simulink library "roller485lib"  (R2023a)
settings: Solver=VariableStepAuto  StartTime=0.0  StopTime=10.0  RelTol=1e-3
libraries: arduinolib x172, simulink x66, $bdroot x1
(part 3 of 5)

== system roller485lib/I2C Write/current command [A] ==
  command [A] : Inport
  A to mA : Gain  Gain=1000
  "Clock " : Clock
  Compare To Constant : simulink/Logic and Bit Operations/Compare To Constant  relop=<=  const=set_time  OutDataTypeStr=boolean
  Data Type Conversion : DataTypeConversion  OutDataTypeStr=uint32  SaturateOnIntegerOverflow=off  RndMeth=Floor
  Enabled Subsystem (mode setting) : $bdroot/I2C Write/current command [mA]/Enabled Subsystem (mode setting)  SystemSampleTime=-1  VariantActivationTime=update diagram  Latency=0  AutoFrameSizeCalculation=off
  I2C Write (0xB0) : arduinolib/I2C Write  I2CModule=0  Mode=Master  SlaveAddress=I2CAddress  SlaveByteOrder=LittleEndian  Direction=Transmitter  RegisterAddressMode=on  RegisterAddress=0xB0  SlaveDataType=uint8  DataLength=1  NoAck=off  RepeatedStart=off  OutputStatus=off  blockPlatform=ARDUINO
  current mode : Constant  Value=3
  x 100 : Gain  Gain=100
  wires:
  x 100/1 -> Data Type Conversion/1
  command [A]/1 -> A to mA/1
  A to mA/1 -> x 100/1
  Data Type Conversion/1 -> I2C Write (0xB0)/1
  Compare To Constant/1 -> Enabled Subsystem (mode setting)/Enable
  current mode/1 -> Enabled Subsystem (mode setting)/1
  "Clock "/1 -> Compare To Constant/1

== system roller485lib/I2C Write/current command [mA] ==
  command [mA] : Inport
  "Clock " : Clock
  Compare To Constant : simulink/Logic and Bit Operations/Compare To Constant  relop=<=  const=set_time  OutDataTypeStr=boolean
  Data Type Conversion : DataTypeConversion  OutDataTypeStr=uint32  SaturateOnIntegerOverflow=off  RndMeth=Floor
  Enabled Subsystem (mode setting) : Subsystem  TreatAsAtomicUnit=on
  I2C Write (0xB0) : arduinolib/I2C Write  I2CModule=0  Mode=Master  SlaveAddress=I2CAddress  SlaveByteOrder=LittleEndian  Direction=Transmitter  RegisterAddressMode=on  RegisterAddress=0xB0  SlaveDataType=uint8  DataLength=1  NoAck=off  RepeatedStart=off  OutputStatus=off  blockPlatform=ARDUINO
  current mode : Constant  Value=3
  x 100 : Gain  Gain=100
  wires:
  current mode/1 -> Enabled Subsystem (mode setting)/1(mode)
  Compare To Constant/1 -> Enabled Subsystem (mode setting)/Enable
  "Clock "/1 -> Compare To Constant/1
  Data Type Conversion/1 -> I2C Write (0xB0)/1
  command [mA]/1 -> x 100/1
  x 100/1 -> Data Type Conversion/1

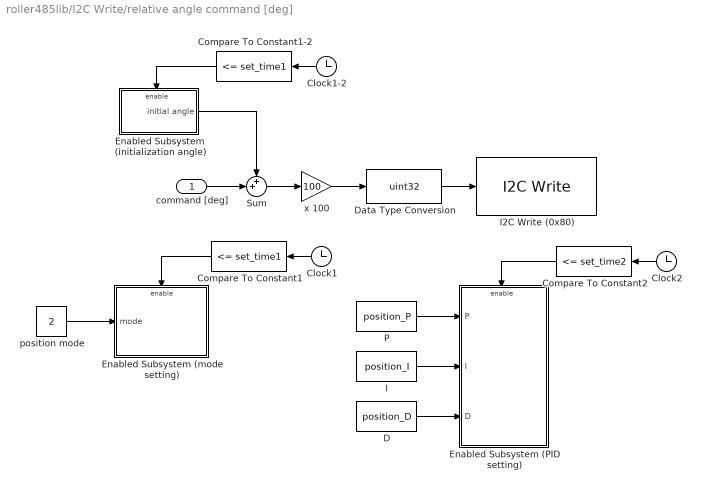
== system roller485lib/I2C Write/relative angle command [deg] ==
  command [deg] : Inport
  Clock1 : Clock
  Clock1-2 : Clock
  Clock2 : Clock
  Compare To Constant1 : simulink/Logic and Bit Operations/Compare To Constant  relop=<=  const=set_time1  OutDataTypeStr=boolean
  Compare To Constant1-2 : simulink/Logic and Bit Operations/Compare To Constant  relop=<=  const=set_time1  OutDataTypeStr=boolean
  Compare To Constant2 : simulink/Logic and Bit Operations/Compare To Constant  relop=<=  const=set_time2  OutDataTypeStr=boolean
  D : Constant  Value=position_D
  Data Type Conversion : DataTypeConversion  OutDataTypeStr=uint32  SaturateOnIntegerOverflow=off  RndMeth=Floor
  Enabled Subsystem (PID setting) : Subsystem  TreatAsAtomicUnit=on
  Enabled Subsystem (initialization angle) : Subsystem  TreatAsAtomicUnit=on
  Enabled Subsystem (mode setting) : Subsystem  TreatAsAtomicUnit=on
  I : Constant  Value=position_I
  I2C Write (0x80) : arduinolib/I2C Write  I2CModule=0  Mode=Master  SlaveAddress=I2CAddress  SlaveByteOrder=LittleEndian  Direction=Transmitter  RegisterAddressMode=on  RegisterAddress=0x80  SlaveDataType=uint8  DataLength=1  NoAck=off  RepeatedStart=off  OutputStatus=off  blockPlatform=ARDUINO
  P : Constant  Value=position_P
  Sum : Sum  Inputs=++|
  position mode : Constant  Value=2
  x 100 : Gain  Gain=100
  wires:
  Compare To Constant1-2/1 -> Enabled Subsystem (initialization angle)/Enable
  command [deg]/1 -> Sum/2
  Enabled Subsystem (initialization angle)/1(initial angle) -> Sum/1
  x 100/1 -> Data Type Conversion/1
  Sum/1 -> x 100/1
  Compare To Constant2/1 -> Enabled Subsystem (PID setting)/Enable
  position mode/1 -> Enabled Subsystem (mode setting)/1(mode)
  P/1 -> Enabled Subsystem (PID setting)/1(P)
  Clock1/1 -> Compare To Constant1/1
  Compare To Constant1/1 -> Enabled Subsystem (mode setting)/Enable
  Data Type Conversion/1 -> I2C Write (0x80)/1
  D/1 -> Enabled Subsystem (PID setting)/3(D)
  I/1 -> Enabled Subsystem (PID setting)/2(I)
  Clock2/1 -> Compare To Constant2/1
  Clock1-2/1 -> Compare To Constant1-2/1

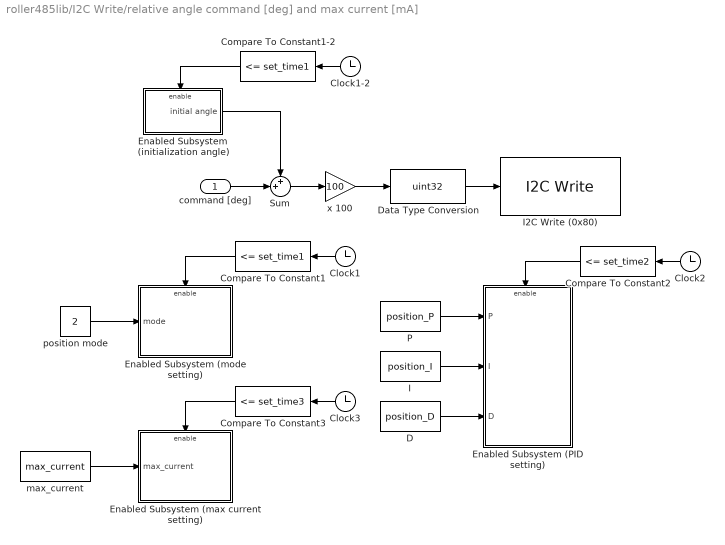
== system roller485lib/I2C Write/relative angle command [deg] and max current [mA] ==
  command [deg] : Inport
  Clock1 : Clock
  Clock1-2 : Clock
  Clock2 : Clock
  Clock3 : Clock
  Compare To Constant1 : simulink/Logic and Bit Operations/Compare To Constant  relop=<=  const=set_time1  OutDataTypeStr=boolean
  Compare To Constant1-2 : simulink/Logic and Bit Operations/Compare To Constant  relop=<=  const=set_time1  OutDataTypeStr=boolean
  Compare To Constant2 : simulink/Logic and Bit Operations/Compare To Constant  relop=<=  const=set_time2  OutDataTypeStr=boolean
  Compare To Constant3 : simulink/Logic and Bit Operations/Compare To Constant  relop=<=  const=set_time3  OutDataTypeStr=boolean
  D : Constant  Value=position_D
  Data Type Conversion : DataTypeConversion  OutDataTypeStr=uint32  SaturateOnIntegerOverflow=off  RndMeth=Floor
  Enabled Subsystem (PID setting) : Subsystem  TreatAsAtomicUnit=on
  Enabled Subsystem (initialization angle) : Subsystem  TreatAsAtomicUnit=on
  Enabled Subsystem (max current setting) : Subsystem  TreatAsAtomicUnit=on
  Enabled Subsystem (mode setting) : Subsystem  TreatAsAtomicUnit=on
  I : Constant  Value=position_I
  I2C Write (0x80) : arduinolib/I2C Write  I2CModule=0  Mode=Master  SlaveAddress=I2CAddress  SlaveByteOrder=LittleEndian  Direction=Transmitter  RegisterAddressMode=on  RegisterAddress=0x80  SlaveDataType=uint8  DataLength=1  NoAck=off  RepeatedStart=off  OutputStatus=off  blockPlatform=ARDUINO
  P : Constant  Value=position_P
  Sum : Sum  Inputs=++|
  max_current : Constant  Value=max_current
  position mode : Constant  Value=2
  x 100 : Gain  Gain=100
  wires:
  Compare To Constant1-2/1 -> Enabled Subsystem (initialization angle)/Enable
  command [deg]/1 -> Sum/2
  Enabled Subsystem (initialization angle)/1(initial angle) -> Sum/1
  x 100/1 -> Data Type Conversion/1
  Sum/1 -> x 100/1
  max_current/1 -> Enabled Subsystem (max current setting)/1(max_current)
  Compare To Constant2/1 -> Enabled Subsystem (PID setting)/Enable
  Compare To Constant3/1 -> Enabled Subsystem (max current setting)/Enable
  position mode/1 -> Enabled Subsystem (mode setting)/1(mode)
  P/1 -> Enabled Subsystem (PID setting)/1(P)
  Clock1/1 -> Compare To Constant1/1
  Compare To Constant1/1 -> Enabled Subsystem (mode setting)/Enable
  Data Type Conversion/1 -> I2C Write (0x80)/1
  D/1 -> Enabled Subsystem (PID setting)/3(D)
  I/1 -> Enabled Subsystem (PID setting)/2(I)
  Clock3/1 -> Compare To Constant3/1
  Clock2/1 -> Compare To Constant2/1
  Clock1-2/1 -> Compare To Constant1-2/1

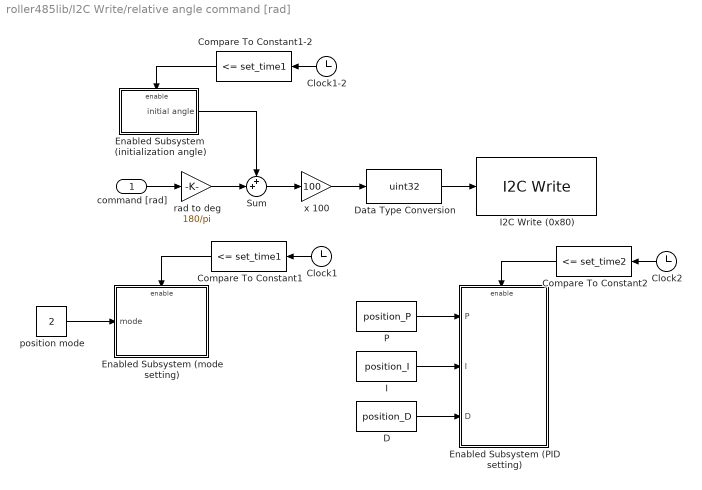
== system roller485lib/I2C Write/relative angle command [rad] ==
  command [rad] : Inport
  Clock1 : Clock
  Clock1-2 : Clock
  Clock2 : Clock
  Compare To Constant1 : simulink/Logic and Bit Operations/Compare To Constant  relop=<=  const=set_time1  OutDataTypeStr=boolean
  Compare To Constant1-2 : simulink/Logic and Bit Operations/Compare To Constant  relop=<=  const=set_time1  OutDataTypeStr=boolean
  Compare To Constant2 : simulink/Logic and Bit Operations/Compare To Constant  relop=<=  const=set_time2  OutDataTypeStr=boolean
  D : Constant  Value=position_D
  Data Type Conversion : DataTypeConversion  OutDataTypeStr=uint32  SaturateOnIntegerOverflow=off  RndMeth=Floor
  Enabled Subsystem (PID setting) : Subsystem  TreatAsAtomicUnit=on
  Enabled Subsystem (initialization angle) : Subsystem  TreatAsAtomicUnit=on
  Enabled Subsystem (mode setting) : Subsystem  TreatAsAtomicUnit=on
  I : Constant  Value=position_I
  I2C Write (0x80) : arduinolib/I2C Write  I2CModule=0  Mode=Master  SlaveAddress=I2CAddress  SlaveByteOrder=LittleEndian  Direction=Transmitter  RegisterAddressMode=on  RegisterAddress=0x80  SlaveDataType=uint8  DataLength=1  NoAck=off  RepeatedStart=off  OutputStatus=off  blockPlatform=ARDUINO
  P : Constant  Value=position_P
  Sum : Sum  Inputs=++|
  position mode : Constant  Value=2
  rad to deg : Gain  Gain=180/pi
  x 100 : Gain  Gain=100
  wires:
  Compare To Constant1-2/1 -> Enabled Subsystem (initialization angle)/Enable
  command [rad]/1 -> rad to deg/1
  rad to deg/1 -> Sum/2
  Enabled Subsystem (initialization angle)/1(initial angle) -> Sum/1
  x 100/1 -> Data Type Conversion/1
  Sum/1 -> x 100/1
  Compare To Constant2/1 -> Enabled Subsystem (PID setting)/Enable
  position mode/1 -> Enabled Subsystem (mode setting)/1(mode)
  P/1 -> Enabled Subsystem (PID setting)/1(P)
  Clock1/1 -> Compare To Constant1/1
  Compare To Constant1/1 -> Enabled Subsystem (mode setting)/Enable
  Data Type Conversion/1 -> I2C Write (0x80)/1
  D/1 -> Enabled Subsystem (PID setting)/3(D)
  I/1 -> Enabled Subsystem (PID setting)/2(I)
  Clock2/1 -> Compare To Constant2/1
  Clock1-2/1 -> Compare To Constant1-2/1

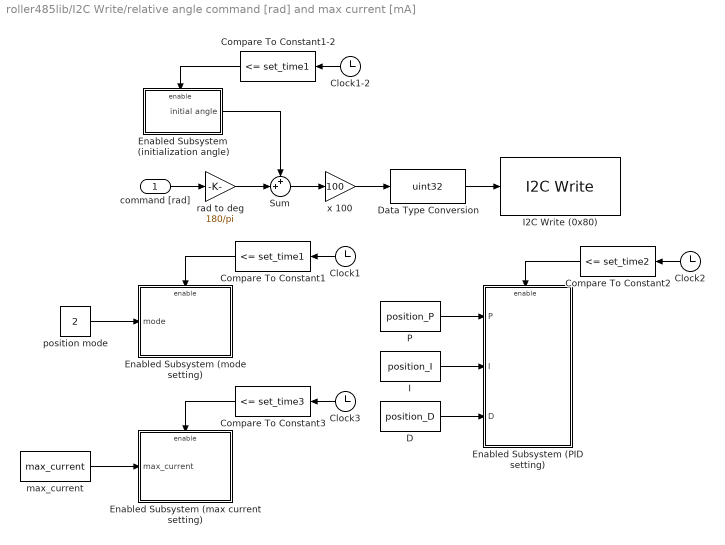
== system roller485lib/I2C Write/relative angle command [rad] and max current [mA] ==
  command [rad] : Inport
  Clock1 : Clock
  Clock1-2 : Clock
  Clock2 : Clock
  Clock3 : Clock
  Compare To Constant1 : simulink/Logic and Bit Operations/Compare To Constant  relop=<=  const=set_time1  OutDataTypeStr=boolean
  Compare To Constant1-2 : simulink/Logic and Bit Operations/Compare To Constant  relop=<=  const=set_time1  OutDataTypeStr=boolean
  Compare To Constant2 : simulink/Logic and Bit Operations/Compare To Constant  relop=<=  const=set_time2  OutDataTypeStr=boolean
  Compare To Constant3 : simulink/Logic and Bit Operations/Compare To Constant  relop=<=  const=set_time3  OutDataTypeStr=boolean
  D : Constant  Value=position_D
  Data Type Conversion : DataTypeConversion  OutDataTypeStr=uint32  SaturateOnIntegerOverflow=off  RndMeth=Floor
  Enabled Subsystem (PID setting) : Subsystem  TreatAsAtomicUnit=on
  Enabled Subsystem (initialization angle) : Subsystem  TreatAsAtomicUnit=on
  Enabled Subsystem (max current setting) : Subsystem  TreatAsAtomicUnit=on
  Enabled Subsystem (mode setting) : Subsystem  TreatAsAtomicUnit=on
  I : Constant  Value=position_I
  I2C Write (0x80) : arduinolib/I2C Write  I2CModule=0  Mode=Master  SlaveAddress=I2CAddress  SlaveByteOrder=LittleEndian  Direction=Transmitter  RegisterAddressMode=on  RegisterAddress=0x80  SlaveDataType=uint8  DataLength=1  NoAck=off  RepeatedStart=off  OutputStatus=off  blockPlatform=ARDUINO
  P : Constant  Value=position_P
  Sum : Sum  Inputs=++|
  max_current : Constant  Value=max_current
  position mode : Constant  Value=2
  rad to deg : Gain  Gain=180/pi
  x 100 : Gain  Gain=100
  wires:
  Enabled Subsystem (initialization angle)/1(initial angle) -> Sum/1
  command [rad]/1 -> rad to deg/1
  x 100/1 -> Data Type Conversion/1
  Sum/1 -> x 100/1
  Data Type Conversion/1 -> I2C Write (0x80)/1
  rad to deg/1 -> Sum/2
  Clock2/1 -> Compare To Constant2/1
  D/1 -> Enabled Subsystem (PID setting)/3(D)
  Compare To Constant1/1 -> Enabled Subsystem (mode setting)/Enable
  I/1 -> Enabled Subsystem (PID setting)/2(I)
  Clock1/1 -> Compare To Constant1/1
  position mode/1 -> Enabled Subsystem (mode setting)/1(mode)
  Compare To Constant3/1 -> Enabled Subsystem (max current setting)/Enable
  Clock3/1 -> Compare To Constant3/1
  P/1 -> Enabled Subsystem (PID setting)/1(P)
  max_current/1 -> Enabled Subsystem (max current setting)/1(max_current)
  Compare To Constant2/1 -> Enabled Subsystem (PID setting)/Enable
  Compare To Constant1-2/1 -> Enabled Subsystem (initialization angle)/Enable
  Clock1-2/1 -> Compare To Constant1-2/1

== system roller485lib/I2C Write (using MATLAB Function)/absolute angle command [deg] (using MATLAB Function) ==
  command [deg] : Inport
  Clock1 : Clock
  Clock2 : Clock
  Compare To Constant1 : simulink/Logic and Bit Operations/Compare To Constant  relop=<=  const=set_time1  OutDataTypeStr=boolean
  Compare To Constant2 : simulink/Logic and Bit Operations/Compare To Constant  relop=<=  const=set_time2  OutDataTypeStr=boolean
  D : Constant  Value=position_D
  Enabled Subsystem (PID setting) : Subsystem  TreatAsAtomicUnit=on
  Enabled Subsystem (mode setting) : Subsystem  TreatAsAtomicUnit=on
  I : Constant  Value=position_I
  I2C Write (0x80) : arduinolib/I2C Write  I2CModule=0  Mode=Master  SlaveAddress=I2CAddress  SlaveByteOrder=BigEndian  Direction=Transmitter  RegisterAddressMode=on  RegisterAddress=0x80  SlaveDataType=uint8  DataLength=1  NoAck=off  RepeatedStart=off  OutputStatus=off  blockPlatform=ARDUINO
  MATLAB Function : MATLAB Function  TreatAsAtomicUnit=on
  P : Constant  Value=position_P
  position mode : Constant  Value=2
  x 100 : Gain  Gain=100
  wires:
  command [deg]/1 -> x 100/1
  x 100/1 -> MATLAB Function/1(double_data)
  D/1 -> Enabled Subsystem (PID setting)/3(D)
  I/1 -> Enabled Subsystem (PID setting)/2(I)
  P/1 -> Enabled Subsystem (PID setting)/1(P)
  position mode/1 -> Enabled Subsystem (mode setting)/1(mode)
  MATLAB Function/1(bytes) -> I2C Write (0x80)/1
  Compare To Constant2/1 -> Enabled Subsystem (PID setting)/Enable
  Clock1/1 -> Compare To Constant1/1
  Clock2/1 -> Compare To Constant2/1
  Compare To Constant1/1 -> Enabled Subsystem (mode setting)/Enable

== system roller485lib/I2C Write (using MATLAB Function)/absolute angle command [rad] (using MATLAB Function) ==
  command [rad] : Inport
  Clock1 : Clock
  Clock2 : Clock
  Compare To Constant1 : simulink/Logic and Bit Operations/Compare To Constant  relop=<=  const=set_time1  OutDataTypeStr=boolean
  Compare To Constant2 : simulink/Logic and Bit Operations/Compare To Constant  relop=<=  const=set_time2  OutDataTypeStr=boolean
  D : Constant  Value=position_D
  Enabled Subsystem (PID setting) : Subsystem  TreatAsAtomicUnit=on
  Enabled Subsystem (mode setting) : Subsystem  TreatAsAtomicUnit=on
  I : Constant  Value=position_I
  I2C Write (0x80) : arduinolib/I2C Write  I2CModule=0  Mode=Master  SlaveAddress=I2CAddress  SlaveByteOrder=BigEndian  Direction=Transmitter  RegisterAddressMode=on  RegisterAddress=0x80  SlaveDataType=uint8  DataLength=1  NoAck=off  RepeatedStart=off  OutputStatus=off  blockPlatform=ARDUINO
  MATLAB Function : MATLAB Function  TreatAsAtomicUnit=on
  P : Constant  Value=position_P
  position mode : Constant  Value=2
  rad to deg : Gain  Gain=180/pi
  x 100 : Gain  Gain=100
  wires:
  position mode/1 -> Enabled Subsystem (mode setting)/1(mode)
  P/1 -> Enabled Subsystem (PID setting)/1(P)
  I/1 -> Enabled Subsystem (PID setting)/2(I)
  D/1 -> Enabled Subsystem (PID setting)/3(D)
  x 100/1 -> MATLAB Function/1(double_data)
  rad to deg/1 -> x 100/1
  command [rad]/1 -> rad to deg/1
  MATLAB Function/1(bytes) -> I2C Write (0x80)/1
  Compare To Constant2/1 -> Enabled Subsystem (PID setting)/Enable
  Clock1/1 -> Compare To Constant1/1
  Clock2/1 -> Compare To Constant2/1
  Compare To Constant1/1 -> Enabled Subsystem (mode setting)/Enable

== system roller485lib/I2C Write (using MATLAB Function)/angular velocity command [rad//s] (using MATLAB Function) ==
  command [rad/s] : Inport
  Clock1 : Clock
  Clock2 : Clock
  Compare To Constant1 : simulink/Logic and Bit Operations/Compare To Constant  relop=<=  const=set_time1  OutDataTypeStr=boolean
  Compare To Constant2 : simulink/Logic and Bit Operations/Compare To Constant  relop=<=  const=set_time2  OutDataTypeStr=boolean
  D : Constant  Value=speed_D
  Enabled Subsystem (PID setting) : Subsystem  TreatAsAtomicUnit=on
  Enabled Subsystem (mode setting) : Subsystem  TreatAsAtomicUnit=on
  I : Constant  Value=speed_I
  I2C Write (0x40) : arduinolib/I2C Write  I2CModule=0  Mode=Master  SlaveAddress=I2CAddress  SlaveByteOrder=BigEndian  Direction=Transmitter  RegisterAddressMode=on  RegisterAddress=0x40  SlaveDataType=uint8  DataLength=1  NoAck=off  RepeatedStart=off  OutputStatus=off  blockPlatform=ARDUINO
  MATLAB Function : MATLAB Function  TreatAsAtomicUnit=on
  P : Constant  Value=speed_P
  rad/s to rpm : Gain  Gain=60/(2*pi)
  speed mode : Constant
  x 100 : Gain  Gain=100
  wires:
  D/1 -> Enabled Subsystem (PID setting)/3(D)
  speed mode/1 -> Enabled Subsystem (mode setting)/1(mode)
  P/1 -> Enabled Subsystem (PID setting)/1(P)
  I/1 -> Enabled Subsystem (PID setting)/2(I)
  x 100/1 -> MATLAB Function/1(double_data)
  rad/s to rpm/1 -> x 100/1
  command [rad/s]/1 -> rad/s to rpm/1
  MATLAB Function/1(bytes) -> I2C Write (0x40)/1
  Compare To Constant2/1 -> Enabled Subsystem (PID setting)/Enable
  Clock1/1 -> Compare To Constant1/1
  Clock2/1 -> Compare To Constant2/1
  Compare To Constant1/1 -> Enabled Subsystem (mode setting)/Enable

== system roller485lib/I2C Write (using MATLAB Function)/angular velocity command [rpm] (using MATLAB Function) ==
  command [rpm] : Inport
  Clock1 : Clock
  Clock2 : Clock
  Compare To Constant1 : simulink/Logic and Bit Operations/Compare To Constant  relop=<=  const=set_time1  OutDataTypeStr=boolean
  Compare To Constant2 : simulink/Logic and Bit Operations/Compare To Constant  relop=<=  const=set_time2  OutDataTypeStr=boolean
  D : Constant  Value=speed_D
  Enabled Subsystem (PID setting) : Subsystem  TreatAsAtomicUnit=on
  Enabled Subsystem (mode setting) : Subsystem  TreatAsAtomicUnit=on
  I : Constant  Value=speed_I
  I2C Write (0x40) : arduinolib/I2C Write  I2CModule=0  Mode=Master  SlaveAddress=I2CAddress  SlaveByteOrder=BigEndian  Direction=Transmitter  RegisterAddressMode=on  RegisterAddress=0x40  SlaveDataType=uint8  DataLength=1  NoAck=off  RepeatedStart=off  OutputStatus=off  blockPlatform=ARDUINO
  MATLAB Function : MATLAB Function  TreatAsAtomicUnit=on
  P : Constant  Value=speed_P
  speed mode : Constant
  x 100 : Gain  Gain=100
  wires:
  command [rpm]/1 -> x 100/1
  x 100/1 -> MATLAB Function/1(double_data)
  I/1 -> Enabled Subsystem (PID setting)/2(I)
  P/1 -> Enabled Subsystem (PID setting)/1(P)
  speed mode/1 -> Enabled Subsystem (mode setting)/1(mode)
  D/1 -> Enabled Subsystem (PID setting)/3(D)
  MATLAB Function/1(bytes) -> I2C Write (0x40)/1
  Compare To Constant2/1 -> Enabled Subsystem (PID setting)/Enable
  Clock1/1 -> Compare To Constant1/1
  Clock2/1 -> Compare To Constant2/1
  Compare To Constant1/1 -> Enabled Subsystem (mode setting)/Enable

== system roller485lib/I2C Write (using MATLAB Function)/current command [A] (using MATLAB Function) ==
  command [A] : Inport
  A to mA : Gain  Gain=1000
  "Clock " : Clock
  Compare To Constant : simulink/Logic and Bit Operations/Compare To Constant  relop=<=  const=set_time  OutDataTypeStr=boolean
  Enabled Subsystem (mode setting) : Subsystem  TreatAsAtomicUnit=on
  I2C Write (0xB0) : arduinolib/I2C Write  I2CModule=0  Mode=Master  SlaveAddress=I2CAddress  SlaveByteOrder=BigEndian  Direction=Transmitter  RegisterAddressMode=on  RegisterAddress=0xB0  SlaveDataType=uint8  DataLength=1  NoAck=off  RepeatedStart=off  OutputStatus=off  blockPlatform=ARDUINO
  MATLAB Function : MATLAB Function  TreatAsAtomicUnit=on
  current mode : Constant  Value=3
  x 100 : Gain  Gain=100
  wires:
  current mode/1 -> Enabled Subsystem (mode setting)/1(mode)
  A to mA/1 -> x 100/1
  command [A]/1 -> A to mA/1
  x 100/1 -> MATLAB Function/1(double_data)
  MATLAB Function/1(bytes) -> I2C Write (0xB0)/1
  Compare To Constant/1 -> Enabled Subsystem (mode setting)/Enable
  "Clock "/1 -> Compare To Constant/1

== system roller485lib/I2C Write (using MATLAB Function)/current command [mA] (using MATLAB Function) ==
  command [mA] : Inport
  "Clock " : Clock
  Compare To Constant : simulink/Logic and Bit Operations/Compare To Constant  relop=<=  const=set_time  OutDataTypeStr=boolean
  Enabled Subsystem (mode setting) : Subsystem  TreatAsAtomicUnit=on
  I2C Write (0xB0) : arduinolib/I2C Write  I2CModule=0  Mode=Master  SlaveAddress=I2CAddress  SlaveByteOrder=BigEndian  Direction=Transmitter  RegisterAddressMode=on  RegisterAddress=0xB0  SlaveDataType=uint8  DataLength=1  NoAck=off  RepeatedStart=off  OutputStatus=off  blockPlatform=ARDUINO
  MATLAB Function : MATLAB Function  TreatAsAtomicUnit=on
  current mode : Constant  Value=3
  x 100 : Gain  Gain=100
  wires:
  x 100/1 -> MATLAB Function/1(double_data)
  command [mA]/1 -> x 100/1
  current mode/1 -> Enabled Subsystem (mode setting)/1(mode)
  MATLAB Function/1(bytes) -> I2C Write (0xB0)/1
  Compare To Constant/1 -> Enabled Subsystem (mode setting)/Enable
  "Clock "/1 -> Compare To Constant/1

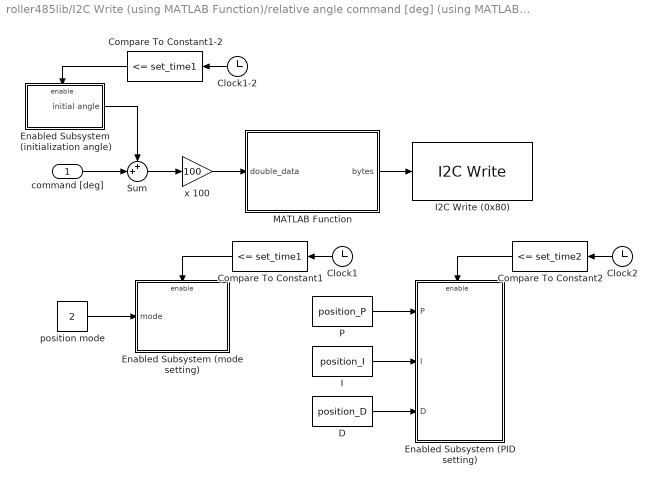
== system roller485lib/I2C Write (using MATLAB Function)/relative angle command [deg] (using MATLAB Function) ==
  command [deg] : Inport
  Clock1 : Clock
  Clock1-2 : Clock
  Clock2 : Clock
  Compare To Constant1 : simulink/Logic and Bit Operations/Compare To Constant  relop=<=  const=set_time1  OutDataTypeStr=boolean
  Compare To Constant1-2 : simulink/Logic and Bit Operations/Compare To Constant  relop=<=  const=set_time1  OutDataTypeStr=boolean
  Compare To Constant2 : simulink/Logic and Bit Operations/Compare To Constant  relop=<=  const=set_time2  OutDataTypeStr=boolean
  D : Constant  Value=position_D
  Enabled Subsystem (PID setting) : Subsystem  TreatAsAtomicUnit=on
  Enabled Subsystem (initialization angle) : Subsystem  TreatAsAtomicUnit=on
  Enabled Subsystem (mode setting) : Subsystem  TreatAsAtomicUnit=on
  I : Constant  Value=position_I
  I2C Write (0x80) : arduinolib/I2C Write  I2CModule=0  Mode=Master  SlaveAddress=I2CAddress  SlaveByteOrder=BigEndian  Direction=Transmitter  RegisterAddressMode=on  RegisterAddress=0x80  SlaveDataType=uint8  DataLength=1  NoAck=off  RepeatedStart=off  OutputStatus=off  blockPlatform=ARDUINO
  MATLAB Function : MATLAB Function  TreatAsAtomicUnit=on
  P : Constant  Value=position_P
  Sum : Sum  Inputs=++|
  position mode : Constant  Value=2
  x 100 : Gain  Gain=100
  wires:
  D/1 -> Enabled Subsystem (PID setting)/3(D)
  Sum/1 -> x 100/1
  Enabled Subsystem (initialization angle)/1(initial angle) -> Sum/1
  command [deg]/1 -> Sum/2
  x 100/1 -> MATLAB Function/1(double_data)
  I/1 -> Enabled Subsystem (PID setting)/2(I)
  P/1 -> Enabled Subsystem (PID setting)/1(P)
  position mode/1 -> Enabled Subsystem (mode setting)/1(mode)
  MATLAB Function/1(bytes) -> I2C Write (0x80)/1
  Clock1/1 -> Compare To Constant1/1
  Clock1-2/1 -> Compare To Constant1-2/1
  Clock2/1 -> Compare To Constant2/1
  Compare To Constant1/1 -> Enabled Subsystem (mode setting)/Enable
  Compare To Constant1-2/1 -> Enabled Subsystem (initialization angle)/Enable
  Compare To Constant2/1 -> Enabled Subsystem (PID setting)/Enable

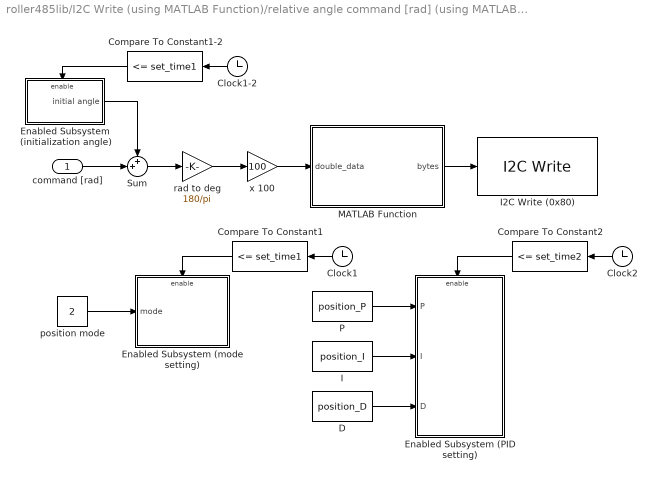
== system roller485lib/I2C Write (using MATLAB Function)/relative angle command [rad] (using MATLAB Function) ==
  command [rad] : Inport
  Clock1 : Clock
  Clock1-2 : Clock
  Clock2 : Clock
  Compare To Constant1 : simulink/Logic and Bit Operations/Compare To Constant  relop=<=  const=set_time1  OutDataTypeStr=boolean
  Compare To Constant1-2 : simulink/Logic and Bit Operations/Compare To Constant  relop=<=  const=set_time1  OutDataTypeStr=boolean
  Compare To Constant2 : simulink/Logic and Bit Operations/Compare To Constant  relop=<=  const=set_time2  OutDataTypeStr=boolean
  D : Constant  Value=position_D
  Enabled Subsystem (PID setting) : Subsystem  TreatAsAtomicUnit=on
  Enabled Subsystem (initialization angle) : Subsystem  TreatAsAtomicUnit=on
  Enabled Subsystem (mode setting) : Subsystem  TreatAsAtomicUnit=on
  I : Constant  Value=position_I
  I2C Write (0x80) : arduinolib/I2C Write  I2CModule=0  Mode=Master  SlaveAddress=I2CAddress  SlaveByteOrder=BigEndian  Direction=Transmitter  RegisterAddressMode=on  RegisterAddress=0x80  SlaveDataType=uint8  DataLength=1  NoAck=off  RepeatedStart=off  OutputStatus=off  blockPlatform=ARDUINO
  MATLAB Function : MATLAB Function  TreatAsAtomicUnit=on
  P : Constant  Value=position_P
  Sum : Sum  Inputs=++|
  position mode : Constant  Value=2
  rad to deg : Gain  Gain=180/pi
  x 100 : Gain  Gain=100
  wires:
  D/1 -> Enabled Subsystem (PID setting)/3(D)
  position mode/1 -> Enabled Subsystem (mode setting)/1(mode)
  P/1 -> Enabled Subsystem (PID setting)/1(P)
  I/1 -> Enabled Subsystem (PID setting)/2(I)
  rad to deg/1 -> x 100/1
  x 100/1 -> MATLAB Function/1(double_data)
  command [rad]/1 -> Sum/2
  Enabled Subsystem (initialization angle)/1(initial angle) -> Sum/1
  Sum/1 -> rad to deg/1
  MATLAB Function/1(bytes) -> I2C Write (0x80)/1
  Clock1/1 -> Compare To Constant1/1
  Clock1-2/1 -> Compare To Constant1-2/1
  Compare To Constant1-2/1 -> Enabled Subsystem (initialization angle)/Enable
  Clock2/1 -> Compare To Constant2/1
  Compare To Constant1/1 -> Enabled Subsystem (mode setting)/Enable
  Compare To Constant2/1 -> Enabled Subsystem (PID setting)/Enable

== system roller485lib/control mode (initial time only)/Enabled Subsystem ==
  mode : Inport
  Enable : EnablePort
  Data Type Conversion : DataTypeConversion  OutDataTypeStr=uint8  SaturateOnIntegerOverflow=off  RndMeth=Floor
  I2C Write (0x01) : arduinolib/I2C Write  I2CModule=0  Mode=Master  SlaveAddress=I2CAddress  SlaveByteOrder=BigEndian  Direction=Transmitter  RegisterAddressMode=on  RegisterAddress=0x01  SlaveDataType=uint8  DataLength=1  NoAck=off  RepeatedStart=off  OutputStatus=off  blockPlatform=ARDUINO
  wires:
  Data Type Conversion/1 -> I2C Write (0x01)/1
  mode/1 -> Data Type Conversion/1

== system roller485lib/Basic I2C Write/basic relative angle command [deg]/Enabled Subsystem (initialization angle) ==
  Enable : EnablePort
  Data Type Conversion : DataTypeConversion  OutDataTypeStr=double  SaturateOnIntegerOverflow=off  RndMeth=Floor
  I2C Read (0x90) : arduinolib/I2C Read  I2CModule=0  Mode=Master  SlaveAddress=I2CAddress  SlaveByteOrder=LittleEndian  Direction=Receiver  RegisterAddressMode=on  RegisterAddress=0x90  SlaveDataType=int32  DataLength=1  NoAck=off  RepeatedStart=off  OutputStatus=off  blockPlatform=ARDUINO  SampleTime=sample_time
  x (1/100) : Gain  Gain=1/100
  initial angle : Outport
  wires:
  I2C Read (0x90)/1 -> Data Type Conversion/1
  Data Type Conversion/1 -> x (1/100)/1
  x (1/100)/1 -> initial angle/1

== system roller485lib/Basic I2C Write/basic relative angle command [rad]/Enabled Subsystem (initialization angle) ==
  Enable : EnablePort
  Data Type Conversion : DataTypeConversion  OutDataTypeStr=double  SaturateOnIntegerOverflow=off  RndMeth=Floor
  I2C Read (0x90) : arduinolib/I2C Read  I2CModule=0  Mode=Master  SlaveAddress=I2CAddress  SlaveByteOrder=LittleEndian  Direction=Receiver  RegisterAddressMode=on  RegisterAddress=0x90  SlaveDataType=int32  DataLength=1  NoAck=off  RepeatedStart=off  OutputStatus=off  blockPlatform=ARDUINO  SampleTime=sample_time
  x (1/100) : Gain  Gain=1/100
  initial angle : Outport
  wires:
  I2C Read (0x90)/1 -> Data Type Conversion/1
  Data Type Conversion/1 -> x (1/100)/1
  x (1/100)/1 -> initial angle/1

== system roller485lib/Basic I2C Write/position PID (within set time)/Enabled Subsystem ==
  P : Inport
  I : Inport  Port=2
  D : Inport  Port=3
  Enable : EnablePort
  " x 10^5 " : Gain  Gain=1e5
  Data Type Conversion1 : DataTypeConversion  OutDataTypeStr=uint32  SaturateOnIntegerOverflow=off  RndMeth=Floor
  Data Type Conversion2 : DataTypeConversion  OutDataTypeStr=uint32  SaturateOnIntegerOverflow=off  RndMeth=Floor
  Data Type Conversion3 : DataTypeConversion  OutDataTypeStr=uint32  SaturateOnIntegerOverflow=off  RndMeth=Floor
  I2C Write (0xA0) : arduinolib/I2C Write  I2CModule=0  Mode=Master  SlaveAddress=I2CAddress  SlaveByteOrder=LittleEndian  Direction=Transmitter  RegisterAddressMode=on  RegisterAddress=0xA0  SlaveDataType=uint8  DataLength=1  NoAck=off  RepeatedStart=off  OutputStatus=off  blockPlatform=ARDUINO
  I2C Write (0xA4) : arduinolib/I2C Write  I2CModule=0  Mode=Master  SlaveAddress=I2CAddress  SlaveByteOrder=LittleEndian  Direction=Transmitter  RegisterAddressMode=on  RegisterAddress=0xA4  SlaveDataType=uint8  DataLength=1  NoAck=off  RepeatedStart=off  OutputStatus=off  blockPlatform=ARDUINO
  I2C Write (0xA8) : arduinolib/I2C Write  I2CModule=0  Mode=Master  SlaveAddress=I2CAddress  SlaveByteOrder=LittleEndian  Direction=Transmitter  RegisterAddressMode=on  RegisterAddress=0xA8  SlaveDataType=uint8  DataLength=1  NoAck=off  RepeatedStart=off  OutputStatus=off  blockPlatform=ARDUINO
  x 10^5 : Gain  Gain=1e5
  x 10^7 : Gain  Gain=1e7
  wires:
  P/1 -> x 10^5/1
  I/1 -> x 10^7/1
  D/1 -> " x 10^5 "/1
  x 10^5/1 -> Data Type Conversion1/1
  x 10^7/1 -> Data Type Conversion2/1
  " x 10^5 "/1 -> Data Type Conversion3/1
  Data Type Conversion3/1 -> I2C Write (0xA8)/1
  Data Type Conversion2/1 -> I2C Write (0xA4)/1
  Data Type Conversion1/1 -> I2C Write (0xA0)/1

== system roller485lib/Basic I2C Write/speed PID (within set time)/Enabled Subsystem ==
  P : Inport
  I : Inport  Port=2
  D : Inport  Port=3
  Enable : EnablePort
  " x 10^5 " : Gain  Gain=1e5
  Data Type Conversion1 : DataTypeConversion  OutDataTypeStr=uint32  SaturateOnIntegerOverflow=off  RndMeth=Floor
  Data Type Conversion2 : DataTypeConversion  OutDataTypeStr=uint32  SaturateOnIntegerOverflow=off  RndMeth=Floor
  Data Type Conversion3 : DataTypeConversion  OutDataTypeStr=uint32  SaturateOnIntegerOverflow=off  RndMeth=Floor
  I2C Write (0x70) : arduinolib/I2C Write  I2CModule=0  Mode=Master  SlaveAddress=I2CAddress  SlaveByteOrder=LittleEndian  Direction=Transmitter  RegisterAddressMode=on  RegisterAddress=0x70  SlaveDataType=uint8  DataLength=1  NoAck=off  RepeatedStart=off  OutputStatus=off  blockPlatform=ARDUINO
  I2C Write (0x74) : arduinolib/I2C Write  I2CModule=0  Mode=Master  SlaveAddress=I2CAddress  SlaveByteOrder=LittleEndian  Direction=Transmitter  RegisterAddressMode=on  RegisterAddress=0x74  SlaveDataType=uint8  DataLength=1  NoAck=off  RepeatedStart=off  OutputStatus=off  blockPlatform=ARDUINO
  I2C Write (0x78) : arduinolib/I2C Write  I2CModule=0  Mode=Master  SlaveAddress=I2CAddress  SlaveByteOrder=LittleEndian  Direction=Transmitter  RegisterAddressMode=on  RegisterAddress=0x78  SlaveDataType=uint8  DataLength=1  NoAck=off  RepeatedStart=off  OutputStatus=off  blockPlatform=ARDUINO
  x 10^5 : Gain  Gain=1e5
  x 10^7 : Gain  Gain=1e7
  wires:
  D/1 -> " x 10^5 "/1
  I/1 -> x 10^7/1
  P/1 -> x 10^5/1
  x 10^5/1 -> Data Type Conversion1/1
  " x 10^5 "/1 -> Data Type Conversion3/1
  x 10^7/1 -> Data Type Conversion2/1
  Data Type Conversion2/1 -> I2C Write (0x74)/1
  Data Type Conversion3/1 -> I2C Write (0x78)/1
  Data Type Conversion1/1 -> I2C Write (0x70)/1

== system roller485lib/Basic I2C Write (using MATLAB Function)/basic relative angle command [deg] (using MATLAB Function)/Enabled Subsystem (initialization angle) ==
  Enable : EnablePort
  I2C Read (0x90) : arduinolib/I2C Read  I2CModule=0  Mode=Master  SlaveAddress=0x64  SlaveByteOrder=BigEndian  Direction=Receiver  RegisterAddressMode=on  RegisterAddress=0x90  SlaveDataType=uint8  DataLength=4  NoAck=off  RepeatedStart=off  OutputStatus=off  blockPlatform=ARDUINO  SampleTime=sample_time
  MATLAB Function : MATLAB Function  TreatAsAtomicUnit=on
  x (1/100) : Gain  Gain=1/100
  initial angle : Outport
  wires:
  MATLAB Function/1(double_data) -> x (1/100)/1
  I2C Read (0x90)/1 -> MATLAB Function/1(bytes)
  x (1/100)/1 -> initial angle/1

== system roller485lib/Basic I2C Write (using MATLAB Function)/basic relative angle command [rad] (using MATLAB Function)/Enabled Subsystem (initialization angle) ==
  Enable : EnablePort
  I2C Read (0x90) : arduinolib/I2C Read  I2CModule=0  Mode=Master  SlaveAddress=0x64  SlaveByteOrder=BigEndian  Direction=Receiver  RegisterAddressMode=on  RegisterAddress=0x90  SlaveDataType=uint8  DataLength=4  NoAck=off  RepeatedStart=off  OutputStatus=off  blockPlatform=ARDUINO  SampleTime=sample_time
  MATLAB Function : MATLAB Function  TreatAsAtomicUnit=on
  x (1/100) : Gain  Gain=1/100
  initial angle : Outport
  wires:
  x (1/100)/1 -> initial angle/1
  I2C Read (0x90)/1 -> MATLAB Function/1(bytes)
  MATLAB Function/1(double_data) -> x (1/100)/1

== system roller485lib/Basic I2C Write (using MATLAB Function)/position PID (within set time) (using MATLAB Function)/Enabled Subsystem ==
  P : Inport
  I : Inport  Port=2
  D : Inport  Port=3
  Enable : EnablePort
  " x 10^5 " : Gain  Gain=1e5
  I2C Write (0xA0) : arduinolib/I2C Write  I2CModule=0  Mode=Master  SlaveAddress=I2CAddress  SlaveByteOrder=BigEndian  Direction=Transmitter  RegisterAddressMode=on  RegisterAddress=0xA0  SlaveDataType=uint8  DataLength=1  NoAck=off  RepeatedStart=off  OutputStatus=off  blockPlatform=ARDUINO
  I2C Write (0xA4) : arduinolib/I2C Write  I2CModule=0  Mode=Master  SlaveAddress=I2CAddress  SlaveByteOrder=BigEndian  Direction=Transmitter  RegisterAddressMode=on  RegisterAddress=0xA4  SlaveDataType=uint8  DataLength=1  NoAck=off  RepeatedStart=off  OutputStatus=off  blockPlatform=ARDUINO
  I2C Write (0xA8) : arduinolib/I2C Write  I2CModule=0  Mode=Master  SlaveAddress=I2CAddress  SlaveByteOrder=BigEndian  Direction=Transmitter  RegisterAddressMode=on  RegisterAddress=0xA8  SlaveDataType=uint8  DataLength=1  NoAck=off  RepeatedStart=off  OutputStatus=off  blockPlatform=ARDUINO
  MATLAB Function (D) : MATLAB Function  TreatAsAtomicUnit=on
  MATLAB Function (I) : MATLAB Function  TreatAsAtomicUnit=on
  MATLAB Function (P) : MATLAB Function  TreatAsAtomicUnit=on
  x 10^5 : Gain  Gain=1e5
  x 10^7 : Gain  Gain=1e7
  wires:
  MATLAB Function (D)/1(bytes) -> I2C Write (0xA8)/1
  x 10^7/1 -> MATLAB Function (I)/1(double_data)
  MATLAB Function (P)/1(bytes) -> I2C Write (0xA0)/1
  " x 10^5 "/1 -> MATLAB Function (D)/1(double_data)
  MATLAB Function (I)/1(bytes) -> I2C Write (0xA4)/1
  x 10^5/1 -> MATLAB Function (P)/1(double_data)
  P/1 -> x 10^5/1
  I/1 -> x 10^7/1
  D/1 -> " x 10^5 "/1

== system roller485lib/Basic I2C Write (using MATLAB Function)/speed PID (within set time) (using MATLAB Function)/Enabled Subsystem ==
  P : Inport
  I : Inport  Port=2
  D : Inport  Port=3
  Enable : EnablePort
  " x 10^5 " : Gain  Gain=1e5
  I2C Write (0x70) : arduinolib/I2C Write  I2CModule=0  Mode=Master  SlaveAddress=I2CAddress  SlaveByteOrder=BigEndian  Direction=Transmitter  RegisterAddressMode=on  RegisterAddress=0x70  SlaveDataType=uint8  DataLength=1  NoAck=off  RepeatedStart=off  OutputStatus=off  blockPlatform=ARDUINO
  I2C Write (0x74) : arduinolib/I2C Write  I2CModule=0  Mode=Master  SlaveAddress=I2CAddress  SlaveByteOrder=BigEndian  Direction=Transmitter  RegisterAddressMode=on  RegisterAddress=0x74  SlaveDataType=uint8  DataLength=1  NoAck=off  RepeatedStart=off  OutputStatus=off  blockPlatform=ARDUINO
  I2C Write (0x78) : arduinolib/I2C Write  I2CModule=0  Mode=Master  SlaveAddress=I2CAddress  SlaveByteOrder=BigEndian  Direction=Transmitter  RegisterAddressMode=on  RegisterAddress=0x78  SlaveDataType=uint8  DataLength=1  NoAck=off  RepeatedStart=off  OutputStatus=off  blockPlatform=ARDUINO
  MATLAB Function (D) : MATLAB Function  TreatAsAtomicUnit=on
  MATLAB Function (I) : MATLAB Function  TreatAsAtomicUnit=on
  MATLAB Function (P) : MATLAB Function  TreatAsAtomicUnit=on
  x 10^5 : Gain  Gain=1e5
  x 10^7 : Gain  Gain=1e7
  wires:
  D/1 -> " x 10^5 "/1
  I/1 -> x 10^7/1
  P/1 -> x 10^5/1
  x 10^5/1 -> MATLAB Function (P)/1(double_data)
  MATLAB Function (I)/1(bytes) -> I2C Write (0x74)/1
  " x 10^5 "/1 -> MATLAB Function (D)/1(double_data)
  MATLAB Function (P)/1(bytes) -> I2C Write (0x70)/1
  x 10^7/1 -> MATLAB Function (I)/1(double_data)
  MATLAB Function (D)/1(bytes) -> I2C Write (0x78)/1

== system roller485lib/I2C Read/relative angle detection [deg]/Enabled Subsystem (initialization of angle) ==
  phim : Inport
  Enable : EnablePort
  phim(0) : Outport
  wires:
  phim/1 -> phim(0)/1

== system roller485lib/I2C Read/relative angle detection [rad]/Enabled Subsystem (initialization of angle) ==
  phim : Inport
  Enable : EnablePort
  phim(0) : Outport
  wires:
  phim/1 -> phim(0)/1

== system roller485lib/I2C Read (using MATLAB Function)/relative angle detection [deg] (using MATLAB Function)/Enabled Subsystem (initialization of angle) ==
  phim : Inport
  Enable : EnablePort
  phim(0) : Outport
  wires:
  phim/1 -> phim(0)/1

== system roller485lib/I2C Read (using MATLAB Function)/relative angle detection [rad] (using MATLAB Function)/Enabled Subsystem (initialization of angle) ==
  phim : Inport
  Enable : EnablePort
  phim(0) : Outport
  wires:
  phim/1 -> phim(0)/1

== system roller485lib/I2C Write/absolute angle command [deg]/Enabled Subsystem (PID setting) ==
  P : Inport
  I : Inport  Port=2
  D : Inport  Port=3
  Enable : EnablePort
  " x 10^5 " : Gain  Gain=1e5
  Data Type Conversion1 : DataTypeConversion  OutDataTypeStr=uint32  SaturateOnIntegerOverflow=off  RndMeth=Floor
  Data Type Conversion2 : DataTypeConversion  OutDataTypeStr=uint32  SaturateOnIntegerOverflow=off  RndMeth=Floor
  Data Type Conversion3 : DataTypeConversion  OutDataTypeStr=uint32  SaturateOnIntegerOverflow=off  RndMeth=Floor
  I2C Write (0x70) : arduinolib/I2C Write  I2CModule=0  Mode=Master  SlaveAddress=I2CAddress  SlaveByteOrder=LittleEndian  Direction=Transmitter  RegisterAddressMode=on  RegisterAddress=0x70  SlaveDataType=uint8  DataLength=1  NoAck=off  RepeatedStart=off  OutputStatus=off  blockPlatform=ARDUINO
  I2C Write (0x74) : arduinolib/I2C Write  I2CModule=0  Mode=Master  SlaveAddress=I2CAddress  SlaveByteOrder=LittleEndian  Direction=Transmitter  RegisterAddressMode=on  RegisterAddress=0x74  SlaveDataType=uint8  DataLength=1  NoAck=off  RepeatedStart=off  OutputStatus=off  blockPlatform=ARDUINO
  I2C Write (0x78) : arduinolib/I2C Write  I2CModule=0  Mode=Master  SlaveAddress=I2CAddress  SlaveByteOrder=LittleEndian  Direction=Transmitter  RegisterAddressMode=on  RegisterAddress=0x78  SlaveDataType=uint8  DataLength=1  NoAck=off  RepeatedStart=off  OutputStatus=off  blockPlatform=ARDUINO
  x 10^5 : Gain  Gain=1e5
  x 10^7 : Gain  Gain=1e7
  wires:
  P/1 -> x 10^5/1
  I/1 -> x 10^7/1
  D/1 -> " x 10^5 "/1
  Data Type Conversion2/1 -> I2C Write (0x74)/1
  Data Type Conversion3/1 -> I2C Write (0x78)/1
  Data Type Conversion1/1 -> I2C Write (0x70)/1
  x 10^5/1 -> Data Type Conversion1/1
  x 10^7/1 -> Data Type Conversion2/1
  " x 10^5 "/1 -> Data Type Conversion3/1

== system roller485lib/I2C Write/absolute angle command [deg]/Enabled Subsystem (mode setting) ==
  mode : Inport
  Enable : EnablePort
  Data Type Conversion : DataTypeConversion  OutDataTypeStr=uint8  SaturateOnIntegerOverflow=off  RndMeth=Floor
  I2C Write (0x01) : arduinolib/I2C Write  I2CModule=0  Mode=Master  SlaveAddress=I2CAddress  SlaveByteOrder=BigEndian  Direction=Transmitter  RegisterAddressMode=on  RegisterAddress=0x01  SlaveDataType=uint8  DataLength=1  NoAck=off  RepeatedStart=off  OutputStatus=off  blockPlatform=ARDUINO
  wires:
  Data Type Conversion/1 -> I2C Write (0x01)/1
  mode/1 -> Data Type Conversion/1

== system roller485lib/I2C Write/absolute angle command [deg] and max current [mA]/Enabled Subsystem (PID setting) ==
  P : Inport
  I : Inport  Port=2
  D : Inport  Port=3
  Enable : EnablePort
  " x 10^5 " : Gain  Gain=1e5
  Data Type Conversion1 : DataTypeConversion  OutDataTypeStr=uint32  SaturateOnIntegerOverflow=off  RndMeth=Floor
  Data Type Conversion2 : DataTypeConversion  OutDataTypeStr=uint32  SaturateOnIntegerOverflow=off  RndMeth=Floor
  Data Type Conversion3 : DataTypeConversion  OutDataTypeStr=uint32  SaturateOnIntegerOverflow=off  RndMeth=Floor
  I2C Write (0x70) : arduinolib/I2C Write  I2CModule=0  Mode=Master  SlaveAddress=I2CAddress  SlaveByteOrder=LittleEndian  Direction=Transmitter  RegisterAddressMode=on  RegisterAddress=0x70  SlaveDataType=uint8  DataLength=1  NoAck=off  RepeatedStart=off  OutputStatus=off  blockPlatform=ARDUINO
  I2C Write (0x74) : arduinolib/I2C Write  I2CModule=0  Mode=Master  SlaveAddress=I2CAddress  SlaveByteOrder=LittleEndian  Direction=Transmitter  RegisterAddressMode=on  RegisterAddress=0x74  SlaveDataType=uint8  DataLength=1  NoAck=off  RepeatedStart=off  OutputStatus=off  blockPlatform=ARDUINO
  I2C Write (0x78) : arduinolib/I2C Write  I2CModule=0  Mode=Master  SlaveAddress=I2CAddress  SlaveByteOrder=LittleEndian  Direction=Transmitter  RegisterAddressMode=on  RegisterAddress=0x78  SlaveDataType=uint8  DataLength=1  NoAck=off  RepeatedStart=off  OutputStatus=off  blockPlatform=ARDUINO
  x 10^5 : Gain  Gain=1e5
  x 10^7 : Gain  Gain=1e7
  wires:
  P/1 -> x 10^5/1
  I/1 -> x 10^7/1
  D/1 -> " x 10^5 "/1
  Data Type Conversion2/1 -> I2C Write (0x74)/1
  Data Type Conversion3/1 -> I2C Write (0x78)/1
  Data Type Conversion1/1 -> I2C Write (0x70)/1
  x 10^5/1 -> Data Type Conversion1/1
  x 10^7/1 -> Data Type Conversion2/1
  " x 10^5 "/1 -> Data Type Conversion3/1

== system roller485lib/I2C Write/absolute angle command [deg] and max current [mA]/Enabled Subsystem (max current setting) ==
  max_current : Inport
  Enable : EnablePort
  Data Type Conversion : DataTypeConversion  OutDataTypeStr=uint32  SaturateOnIntegerOverflow=off  RndMeth=Floor
  I2C Write (0x50) : arduinolib/I2C Write  I2CModule=0  Mode=Master  SlaveAddress=I2CAddress  SlaveByteOrder=LittleEndian  Direction=Transmitter  RegisterAddressMode=on  RegisterAddress=0x50  SlaveDataType=uint8  DataLength=1  NoAck=off  RepeatedStart=off  OutputStatus=off  blockPlatform=ARDUINO
  x 100 : Gain  Gain=100
  wires:
  x 100/1 -> Data Type Conversion/1
  max_current/1 -> x 100/1
  Data Type Conversion/1 -> I2C Write (0x50)/1

== system roller485lib/I2C Write/absolute angle command [deg] and max current [mA]/Enabled Subsystem (mode setting) ==
  mode : Inport
  Enable : EnablePort
  Data Type Conversion : DataTypeConversion  OutDataTypeStr=uint8  SaturateOnIntegerOverflow=off  RndMeth=Floor
  I2C Write (0x01) : arduinolib/I2C Write  I2CModule=0  Mode=Master  SlaveAddress=I2CAddress  SlaveByteOrder=BigEndian  Direction=Transmitter  RegisterAddressMode=on  RegisterAddress=0x01  SlaveDataType=uint8  DataLength=1  NoAck=off  RepeatedStart=off  OutputStatus=off  blockPlatform=ARDUINO
  wires:
  Data Type Conversion/1 -> I2C Write (0x01)/1
  mode/1 -> Data Type Conversion/1

== system roller485lib/I2C Write/absolute angle command [rad]/Enabled Subsystem (PID setting) ==
  P : Inport
  I : Inport  Port=2
  D : Inport  Port=3
  Enable : EnablePort
  " x 10^5 " : Gain  Gain=1e5
  Data Type Conversion1 : DataTypeConversion  OutDataTypeStr=uint32  SaturateOnIntegerOverflow=off  RndMeth=Floor
  Data Type Conversion2 : DataTypeConversion  OutDataTypeStr=uint32  SaturateOnIntegerOverflow=off  RndMeth=Floor
  Data Type Conversion3 : DataTypeConversion  OutDataTypeStr=uint32  SaturateOnIntegerOverflow=off  RndMeth=Floor
  I2C Write (0x70) : arduinolib/I2C Write  I2CModule=0  Mode=Master  SlaveAddress=I2CAddress  SlaveByteOrder=LittleEndian  Direction=Transmitter  RegisterAddressMode=on  RegisterAddress=0x70  SlaveDataType=uint8  DataLength=1  NoAck=off  RepeatedStart=off  OutputStatus=off  blockPlatform=ARDUINO
  I2C Write (0x74) : arduinolib/I2C Write  I2CModule=0  Mode=Master  SlaveAddress=I2CAddress  SlaveByteOrder=LittleEndian  Direction=Transmitter  RegisterAddressMode=on  RegisterAddress=0x74  SlaveDataType=uint8  DataLength=1  NoAck=off  RepeatedStart=off  OutputStatus=off  blockPlatform=ARDUINO
  I2C Write (0x78) : arduinolib/I2C Write  I2CModule=0  Mode=Master  SlaveAddress=I2CAddress  SlaveByteOrder=LittleEndian  Direction=Transmitter  RegisterAddressMode=on  RegisterAddress=0x78  SlaveDataType=uint8  DataLength=1  NoAck=off  RepeatedStart=off  OutputStatus=off  blockPlatform=ARDUINO
  x 10^5 : Gain  Gain=1e5
  x 10^7 : Gain  Gain=1e7
  wires:
  P/1 -> x 10^5/1
  I/1 -> x 10^7/1
  D/1 -> " x 10^5 "/1
  Data Type Conversion2/1 -> I2C Write (0x74)/1
  Data Type Conversion3/1 -> I2C Write (0x78)/1
  Data Type Conversion1/1 -> I2C Write (0x70)/1
  x 10^5/1 -> Data Type Conversion1/1
  x 10^7/1 -> Data Type Conversion2/1
  " x 10^5 "/1 -> Data Type Conversion3/1

== system roller485lib/I2C Write/absolute angle command [rad]/Enabled Subsystem (mode setting) ==
  mode : Inport
  Enable : EnablePort
  Data Type Conversion : DataTypeConversion  OutDataTypeStr=uint8  SaturateOnIntegerOverflow=off  RndMeth=Floor
  I2C Write (0x01) : arduinolib/I2C Write  I2CModule=0  Mode=Master  SlaveAddress=I2CAddress  SlaveByteOrder=BigEndian  Direction=Transmitter  RegisterAddressMode=on  RegisterAddress=0x01  SlaveDataType=uint8  DataLength=1  NoAck=off  RepeatedStart=off  OutputStatus=off  blockPlatform=ARDUINO
  wires:
  Data Type Conversion/1 -> I2C Write (0x01)/1
  mode/1 -> Data Type Conversion/1

== system roller485lib/I2C Write/absolute angle command [rad] and max current [mA]/Enabled Subsystem (PID setting) ==
  P : Inport
  I : Inport  Port=2
  D : Inport  Port=3
  Enable : EnablePort
  " x 10^5 " : Gain  Gain=1e5
  Data Type Conversion1 : DataTypeConversion  OutDataTypeStr=uint32  SaturateOnIntegerOverflow=off  RndMeth=Floor
  Data Type Conversion2 : DataTypeConversion  OutDataTypeStr=uint32  SaturateOnIntegerOverflow=off  RndMeth=Floor
  Data Type Conversion3 : DataTypeConversion  OutDataTypeStr=uint32  SaturateOnIntegerOverflow=off  RndMeth=Floor
  I2C Write (0x70) : arduinolib/I2C Write  I2CModule=0  Mode=Master  SlaveAddress=I2CAddress  SlaveByteOrder=LittleEndian  Direction=Transmitter  RegisterAddressMode=on  RegisterAddress=0x70  SlaveDataType=uint8  DataLength=1  NoAck=off  RepeatedStart=off  OutputStatus=off  blockPlatform=ARDUINO
  I2C Write (0x74) : arduinolib/I2C Write  I2CModule=0  Mode=Master  SlaveAddress=I2CAddress  SlaveByteOrder=LittleEndian  Direction=Transmitter  RegisterAddressMode=on  RegisterAddress=0x74  SlaveDataType=uint8  DataLength=1  NoAck=off  RepeatedStart=off  OutputStatus=off  blockPlatform=ARDUINO
  I2C Write (0x78) : arduinolib/I2C Write  I2CModule=0  Mode=Master  SlaveAddress=I2CAddress  SlaveByteOrder=LittleEndian  Direction=Transmitter  RegisterAddressMode=on  RegisterAddress=0x78  SlaveDataType=uint8  DataLength=1  NoAck=off  RepeatedStart=off  OutputStatus=off  blockPlatform=ARDUINO
  x 10^5 : Gain  Gain=1e5
  x 10^7 : Gain  Gain=1e7
  wires:
  P/1 -> x 10^5/1
  I/1 -> x 10^7/1
  D/1 -> " x 10^5 "/1
  Data Type Conversion2/1 -> I2C Write (0x74)/1
  Data Type Conversion3/1 -> I2C Write (0x78)/1
  Data Type Conversion1/1 -> I2C Write (0x70)/1
  x 10^5/1 -> Data Type Conversion1/1
  x 10^7/1 -> Data Type Conversion2/1
  " x 10^5 "/1 -> Data Type Conversion3/1

== system roller485lib/I2C Write/absolute angle command [rad] and max current [mA]/Enabled Subsystem (max current setting) ==
  max_current : Inport
  Enable : EnablePort
  Data Type Conversion : DataTypeConversion  OutDataTypeStr=uint32  SaturateOnIntegerOverflow=off  RndMeth=Floor
  I2C Write (0x50) : arduinolib/I2C Write  I2CModule=0  Mode=Master  SlaveAddress=I2CAddress  SlaveByteOrder=LittleEndian  Direction=Transmitter  RegisterAddressMode=on  RegisterAddress=0x50  SlaveDataType=uint8  DataLength=1  NoAck=off  RepeatedStart=off  OutputStatus=off  blockPlatform=ARDUINO
  x 100 : Gain  Gain=100
  wires:
  x 100/1 -> Data Type Conversion/1
  max_current/1 -> x 100/1
  Data Type Conversion/1 -> I2C Write (0x50)/1

== system roller485lib/I2C Write/absolute angle command [rad] and max current [mA]/Enabled Subsystem (mode setting) ==
  mode : Inport
  Enable : EnablePort
  Data Type Conversion : DataTypeConversion  OutDataTypeStr=uint8  SaturateOnIntegerOverflow=off  RndMeth=Floor
  I2C Write (0x01) : arduinolib/I2C Write  I2CModule=0  Mode=Master  SlaveAddress=I2CAddress  SlaveByteOrder=BigEndian  Direction=Transmitter  RegisterAddressMode=on  RegisterAddress=0x01  SlaveDataType=uint8  DataLength=1  NoAck=off  RepeatedStart=off  OutputStatus=off  blockPlatform=ARDUINO
  wires:
  Data Type Conversion/1 -> I2C Write (0x01)/1
  mode/1 -> Data Type Conversion/1

== system roller485lib/I2C Write/angular velocity command [rad//s]/Enabled Subsystem (PID setting) ==
  P : Inport
  I : Inport  Port=2
  D : Inport  Port=3
  Enable : EnablePort
  " x 10^5 " : Gain  Gain=1e5
  Data Type Conversion1 : DataTypeConversion  OutDataTypeStr=uint32  SaturateOnIntegerOverflow=off  RndMeth=Floor
  Data Type Conversion2 : DataTypeConversion  OutDataTypeStr=uint32  SaturateOnIntegerOverflow=off  RndMeth=Floor
  Data Type Conversion3 : DataTypeConversion  OutDataTypeStr=uint32  SaturateOnIntegerOverflow=off  RndMeth=Floor
  I2C Write (0x70) : arduinolib/I2C Write  I2CModule=0  Mode=Master  SlaveAddress=I2CAddress  SlaveByteOrder=LittleEndian  Direction=Transmitter  RegisterAddressMode=on  RegisterAddress=0x70  SlaveDataType=uint8  DataLength=1  NoAck=off  RepeatedStart=off  OutputStatus=off  blockPlatform=ARDUINO
  I2C Write (0x74) : arduinolib/I2C Write  I2CModule=0  Mode=Master  SlaveAddress=I2CAddress  SlaveByteOrder=LittleEndian  Direction=Transmitter  RegisterAddressMode=on  RegisterAddress=0x74  SlaveDataType=uint8  DataLength=1  NoAck=off  RepeatedStart=off  OutputStatus=off  blockPlatform=ARDUINO
  I2C Write (0x78) : arduinolib/I2C Write  I2CModule=0  Mode=Master  SlaveAddress=I2CAddress  SlaveByteOrder=LittleEndian  Direction=Transmitter  RegisterAddressMode=on  RegisterAddress=0x78  SlaveDataType=uint8  DataLength=1  NoAck=off  RepeatedStart=off  OutputStatus=off  blockPlatform=ARDUINO
  x 10^5 : Gain  Gain=1e5
  x 10^7 : Gain  Gain=1e7
  wires:
  P/1 -> x 10^5/1
  I/1 -> x 10^7/1
  D/1 -> " x 10^5 "/1
  Data Type Conversion2/1 -> I2C Write (0x74)/1
  Data Type Conversion3/1 -> I2C Write (0x78)/1
  Data Type Conversion1/1 -> I2C Write (0x70)/1
  x 10^5/1 -> Data Type Conversion1/1
  x 10^7/1 -> Data Type Conversion2/1
  " x 10^5 "/1 -> Data Type Conversion3/1
